simulink model "afe_abc_inv_pmsm"  (R2024b)
settings: Solver=ode1be  StartTime=0.0  StopTime=simlength  FixedStep=tc  MaxStep=tc
undefined symbols (not defined in the file): Adrso, Amplitude_U, Amplitude_V, Amplitude_W, Aresd, b, Bresd, Cresd, Crso, CTRPIFF_CLIP_RELEASE, dead_time_AFE, dead_time_INV, deepNEGeta, deepNEGxi, deepPOSxi, emf_fb_p, emf_fb_p_ccaller_1, emf_fb_p_ccaller_2, emf_p, emf_p_ccaller_1, emf_p_ccaller_2, end_time_LVRT, fPWM_AFE, fPWM_INV, g0_161Hz, g0_500Hz, g1_161Hz, g1_500Hz, i_grid_neg_eta_lim, i_grid_neg_eta_red_lim, i_grid_neg_xi_lim, i_grid_neg_xi_red_lim, i_grid_pos_eta_lim, i_grid_pos_eta_red_lim, ibez, id_lim, ieta_neg_ref_lim, ieta_pos_ref_lim, Igrid_phase_normalization_factor, iq_lim, ixi_pos_ref_lim, Jm, k_frt_ref, kg, ki_afe, ki_i, ki_rc_neg_grid, ki_rc_pos_grid, ki_vs, ki_w, kp_afe, kp_i, kp_rc_neg_grid, kp_rc_pos_grid, kp_vs, kp_w, kw, l1, l2, Ld_norm ... (+45)
libraries: fl_lib x115, nesl_utility x75, cstblocks x14, simulink x13, single_phase_transformer_lib x3, threephase_inductor_lib x2, flexshaft_lib x1, pmsm_uvw_with_harmonics_lib x1
(part 4 of 10)

== system afe_abc_inv_pmsm/afe_abc_inv_psm_mod1/inverter_control/torque_reference ==
  rotor speed : Inport
  1-D Lookup Table : Lookup_n-D  NumberOfTableDimensions=1  BreakpointsForDimension1=rpm_base  Table=torque_base  InternalRulePriority=Speed  RndMeth=Simplest
  Gain : Gain  Gain=-1
  Gain1 : Gain  Gain=1/tau_bez
  Gain2 : Gain  Gain=rpm_bez
  Saturation : Saturate  UpperLimit=0  LowerLimit=-inf
  Transfer Fcn : TransferFcn  Denominator=[1E-4 1]
  torque_ref : Outport
  wires:
  Transfer Fcn/1 -> Gain2/1
  rotor speed/1 -> Transfer Fcn/1
  Gain/1 -> Saturation/1
  Saturation/1 -> torque_ref/1
  Gain1/1 -> Gain/1
  1-D Lookup Table/1 -> Gain1/1
  Gain2/1 -> 1-D Lookup Table/1

== system afe_abc_inv_pmsm/grid/grid_emulator/3ph_Dyg ==
  Electrical Reference1 : fl_lib/Electrical/Electrical Elements/Electrical Reference
  ph1 : single_phase_transformer_lib/single phase transformer  Lm=Lmu2_trafo H  n1=50*sqrt(3)  n2=50  Rd1=0 Ohm  Rd2=Rd2_trafo Ohm  Ld1=0 H  Ld2=Ld2_trafo H  Rfe=Rm2_trafo Ohm  phi_specify=off  phi_priority=None  phi=0 V*s  phi_nominal_specify=off  phi_nominal_unit=V*s  phi_nominal_value=1  i1_specify=off  i1_priority=None  i1=0 A  i1_nominal_specify=off  i1_nominal_unit=A  i1_nominal_value=1  i2_specify=off  i2_priority=None  i2=0 A  i2_nominal_specify=off  i2_nominal_unit=A  i2_nominal_value=1  ife_specify=off  ife_priority=None  ife=0 A  ife_nominal_specify=off  ife_nominal_unit=A  ife_nominal_value=1  u1_specify=off  u1_priority=None  u1=0 V  u1_nominal_specify=off  u1_nominal_unit=V  u1_nominal_value=1  u2_specify=off  u2_priority=None  u2=0 V  u2_nominal_specify=off  u2_nominal_unit=V  u2_nominal_value=1
      settings: InternalSimscapePortConfiguration="{\"Bottom\":[],\"Left\":[{\"id\":\"u1_p\",\"label\":\"u1(+)\",\"type\":\"foundation.electrical.electrical\"},{\"id\":\"u1_n\",\"label\":\"u1(-)\",\"type\":\"foundation.electrical.electrical\"}],\"Right\":[{\"id\":\"u2_p\",\"label\":\"u2(+)\",\"type\":\"foundation.electrical.electrical\"},{\"id\":\"u2_n\",\"label\":\"u2(-)\",\"type\":\"foundation.electrical.electrical\"}],\"Top\":[]}"
  ph2 : single_phase_transformer_lib/single phase transformer  Lm=Lmu2_trafo H  n1=50*sqrt(3)  n2=50  Rd1=0 Ohm  Rd2=Rd2_trafo Ohm  Ld1=0 H  Ld2=Ld2_trafo H  Rfe=Rm2_trafo Ohm  phi_specify=off  phi_priority=None  phi=0 V*s  phi_nominal_specify=off  phi_nominal_unit=V*s  phi_nominal_value=1  i1_specify=off  i1_priority=None  i1=0 A  i1_nominal_specify=off  i1_nominal_unit=A  i1_nominal_value=1  i2_specify=off  i2_priority=None  i2=0 A  i2_nominal_specify=off  i2_nominal_unit=A  i2_nominal_value=1  ife_specify=off  ife_priority=None  ife=0 A  ife_nominal_specify=off  ife_nominal_unit=A  ife_nominal_value=1  u1_specify=off  u1_priority=None  u1=0 V  u1_nominal_specify=off  u1_nominal_unit=V  u1_nominal_value=1  u2_specify=off  u2_priority=None  u2=0 V  u2_nominal_specify=off  u2_nominal_unit=V  u2_nominal_value=1
      settings: InternalSimscapePortConfiguration="{\"Bottom\":[],\"Left\":[{\"id\":\"u1_p\",\"label\":\"u1(+)\",\"type\":\"foundation.electrical.electrical\"},{\"id\":\"u1_n\",\"label\":\"u1(-)\",\"type\":\"foundation.electrical.electrical\"}],\"Right\":[{\"id\":\"u2_p\",\"label\":\"u2(+)\",\"type\":\"foundation.electrical.electrical\"},{\"id\":\"u2_n\",\"label\":\"u2(-)\",\"type\":\"foundation.electrical.electrical\"}],\"Top\":[]}"
  ph3 : single_phase_transformer_lib/single phase transformer  Lm=Lmu2_trafo H  n1=50*sqrt(3)  n2=50  Rd1=0 Ohm  Rd2=Rd2_trafo Ohm  Ld1=0 H  Ld2=Ld2_trafo H  Rfe=Rm2_trafo Ohm  phi_specify=off  phi_priority=None  phi=0 V*s  phi_nominal_specify=off  phi_nominal_unit=V*s  phi_nominal_value=1  i1_specify=off  i1_priority=None  i1=0 A  i1_nominal_specify=off  i1_nominal_unit=A  i1_nominal_value=1  i2_specify=off  i2_priority=None  i2=0 A  i2_nominal_specify=off  i2_nominal_unit=A  i2_nominal_value=1  ife_specify=off  ife_priority=None  ife=0 A  ife_nominal_specify=off  ife_nominal_unit=A  ife_nominal_value=1  u1_specify=off  u1_priority=None  u1=0 V  u1_nominal_specify=off  u1_nominal_unit=V  u1_nominal_value=1  u2_specify=off  u2_priority=None  u2=0 V  u2_nominal_specify=off  u2_nominal_unit=V  u2_nominal_value=1
      settings: InternalSimscapePortConfiguration="{\"Bottom\":[],\"Left\":[{\"id\":\"u1_p\",\"label\":\"u1(+)\",\"type\":\"foundation.electrical.electrical\"},{\"id\":\"u1_n\",\"label\":\"u1(-)\",\"type\":\"foundation.electrical.electrical\"}],\"Right\":[{\"id\":\"u2_p\",\"label\":\"u2(+)\",\"type\":\"foundation.electrical.electrical\"},{\"id\":\"u2_n\",\"label\":\"u2(-)\",\"type\":\"foundation.electrical.electrical\"}],\"Top\":[]}"
  ua : PMIOPort  Side=Right
  ub : PMIOPort  Port=2  Side=Right
  uc : PMIOPort  Port=3  Side=Right
  Ua : PMIOPort  Port=4  Side=Left
  Ub : PMIOPort  Port=5  Side=Left
  Uc : PMIOPort  Port=6  Side=Left
  connections:
  Electrical Reference1/LConn1 -- ph3/RConn2 -- ph2/RConn2 -- ph1/RConn2
  ph3/RConn1 -- uc/RConn1
  ph1/LConn1 -- ph3/LConn2 -- Ua/RConn1
  ph1/RConn1 -- ua/RConn1
  ph2/RConn1 -- ub/RConn1
  ph1/LConn2 -- ph2/LConn1 -- Ub/RConn1
  Uc/RConn1 -- ph3/LConn1 -- ph2/LConn2

== system afe_abc_inv_pmsm/grid/grid_emulator/breaker ==
  PS Step : fl_lib/Physical Signals/Sources/PS Step  step_time=start_time_grid_switch_open s  initial_value=15  final_value=0
  switch_1 : Subsystem
      settings: PortSchema="{\"entries\":[{\"content\":{\"sides\":[{\"content\":{\"connectorIds\":[\"LConn1\"]},\"type\":\"ConnectorPlacement.EquallySpacedRectSide\",\"uuid\":\"9277da8d-d460-43e6-8478-dd662f15d226\"},{\"content\":{\"connectorIds\":[],\"side\":\"RIGHT\"},\"type\":\"ConnectorPlacement.EquallySpacedRectSide\",\"uuid\":\"a7ece396-f1d9-4f4f-a05b-db1fc65d6e1d\"},{\"content\":{\"connectorIds\":[\"LConn2\"],\"side\":\"TOP\"},\"type\":\"ConnectorPlacement.EquallySpacedRectSide\",\"uuid\":\"fdd70777-e9cf-4317-afb6-cae87f75d5b0\"},{\"content\":{\"connectorIds\":[\"RConn1\"],\"side\":\"BOTTOM\"},\"type\":\"ConnectorPlacement.EquallySpacedRectSide\",\"uuid\":\"2353ed68-b1a1-4775-9ca9-31e268d5443b\"}]},\"type\":\"ConnectorPlacement.EquallySpacedConnector\",\"uuid\":\"d5479f4c-4e65-4791-adcb-73df11f88590\"}],\"packageUris\":[\"http://schema.mathworks.com/mf0/Connector/R2020b\"],\"version\":\"1.0\"}"
  switch_2 : Subsystem
      settings: PortSchema="{\"entries\":[{\"content\":{\"sides\":[{\"content\":{\"connectorIds\":[\"LConn1\"]},\"type\":\"ConnectorPlacement.EquallySpacedRectSide\",\"uuid\":\"9277da8d-d460-43e6-8478-dd662f15d226\"},{\"content\":{\"connectorIds\":[],\"side\":\"RIGHT\"},\"type\":\"ConnectorPlacement.EquallySpacedRectSide\",\"uuid\":\"a7ece396-f1d9-4f4f-a05b-db1fc65d6e1d\"},{\"content\":{\"connectorIds\":[\"LConn2\"],\"side\":\"TOP\"},\"type\":\"ConnectorPlacement.EquallySpacedRectSide\",\"uuid\":\"fdd70777-e9cf-4317-afb6-cae87f75d5b0\"},{\"content\":{\"connectorIds\":[\"RConn1\"],\"side\":\"BOTTOM\"},\"type\":\"ConnectorPlacement.EquallySpacedRectSide\",\"uuid\":\"2353ed68-b1a1-4775-9ca9-31e268d5443b\"}]},\"type\":\"ConnectorPlacement.EquallySpacedConnector\",\"uuid\":\"d5479f4c-4e65-4791-adcb-73df11f88590\"}],\"packageUris\":[\"http://schema.mathworks.com/mf0/Connector/R2020b\"],\"version\":\"1.0\"}"
  switch_3 : Subsystem
      settings: PortSchema="{\"entries\":[{\"content\":{\"sides\":[{\"content\":{\"connectorIds\":[\"LConn1\"]},\"type\":\"ConnectorPlacement.EquallySpacedRectSide\",\"uuid\":\"9277da8d-d460-43e6-8478-dd662f15d226\"},{\"content\":{\"connectorIds\":[],\"side\":\"RIGHT\"},\"type\":\"ConnectorPlacement.EquallySpacedRectSide\",\"uuid\":\"a7ece396-f1d9-4f4f-a05b-db1fc65d6e1d\"},{\"content\":{\"connectorIds\":[\"LConn2\"],\"side\":\"TOP\"},\"type\":\"ConnectorPlacement.EquallySpacedRectSide\",\"uuid\":\"fdd70777-e9cf-4317-afb6-cae87f75d5b0\"},{\"content\":{\"connectorIds\":[\"RConn1\"],\"side\":\"BOTTOM\"},\"type\":\"ConnectorPlacement.EquallySpacedRectSide\",\"uuid\":\"2353ed68-b1a1-4775-9ca9-31e268d5443b\"}]},\"type\":\"ConnectorPlacement.EquallySpacedConnector\",\"uuid\":\"d5479f4c-4e65-4791-adcb-73df11f88590\"}],\"packageUris\":[\"http://schema.mathworks.com/mf0/Connector/R2020b\"],\"version\":\"1.0\"}"
  ua : PMIOPort  Side=Right
  Ua : PMIOPort  Port=2  Side=Left
  ub : PMIOPort  Port=3  Side=Right
  Ub : PMIOPort  Port=4  Side=Left
  uc : PMIOPort  Port=5  Side=Right
  Uc : PMIOPort  Port=6  Side=Left
  connections:
  Ub/RConn1 -- switch_2/LConn2
  Uc/RConn1 -- switch_3/LConn2
  Ua/RConn1 -- switch_1/LConn2
  PS Step/RConn1 -- switch_1/LConn1 -- switch_2/LConn1 -- switch_3/LConn1
  switch_1/RConn1 -- ua/RConn1
  ub/RConn1 -- switch_2/RConn1
  switch_3/RConn1 -- uc/RConn1

== system afe_abc_inv_pmsm/grid/grid_emulator/grid_emulator ==
  phase_gen : Subsystem
  voltage_reference : Subsystem
  voltage_source : Subsystem
  Vma : Outport
  Vmb : Outport  Port=2
  Vmc : Outport  Port=3
  wires:
  phase_gen/1(grid_emu_phase) -> voltage_reference/1(grid_emu_phase)  "grid_emu_phase"
  voltage_source/2(vn_xi) -> voltage_reference/3(Vxi_n)
  voltage_source/1(vp_xi) -> voltage_reference/2(Vxi_p)
  voltage_source/3(vn_eta) -> voltage_reference/4(Veta_n)
  voltage_reference/3(V3_ref) -> Vmc/1
  voltage_reference/1(V1_ref) -> Vma/1
  voltage_reference/2(V2_ref) -> Vmb/1

== system afe_abc_inv_pmsm/grid/grid_emulator/threephase_vi_measures ==
  Bus Creator : BusCreator  Inputs=6
  Current Sensor : fl_lib/Electrical/Electrical Sensors/Current Sensor
  Current Sensor1 : fl_lib/Electrical/Electrical Sensors/Current Sensor
  Current Sensor2 : fl_lib/Electrical/Electrical Sensors/Current Sensor
  Electrical Reference1 : fl_lib/Electrical/Electrical Elements/Electrical Reference
  Voltage Sensor : fl_lib/Electrical/Electrical Sensors/Voltage Sensor
  Voltage Sensor1 : fl_lib/Electrical/Electrical Sensors/Voltage Sensor
  Voltage Sensor2 : fl_lib/Electrical/Electrical Sensors/Voltage Sensor
  i : Selector  InputPortWidth=6  IndexOptions=Index vector (dialog)  Indices=[4 5 6]  OutputSizes=1
  i_line_abc/u_line_abc : Scope  NumInputPorts=2
  ia_grid : nesl_utility/PS-Simulink Converter  PhysicalDomain=network_engine_domain  SubClassName=ps_output  LeftPortType=input  RightPortType=output  PseudoPeriodic=off  Frequencies=[]  VectorFormat=1-D array  Unit=A  AffineConversion=off
  ib_grid : nesl_utility/PS-Simulink Converter  PhysicalDomain=network_engine_domain  SubClassName=ps_output  LeftPortType=input  RightPortType=output  PseudoPeriodic=off  Frequencies=[]  VectorFormat=1-D array  Unit=A  AffineConversion=off
  ic_grid : nesl_utility/PS-Simulink Converter  PhysicalDomain=network_engine_domain  SubClassName=ps_output  LeftPortType=input  RightPortType=output  PseudoPeriodic=off  Frequencies=[]  VectorFormat=1-D array  Unit=A  AffineConversion=off
  u : Selector  InputPortWidth=6  IndexOptions=Index vector (dialog)  Indices=[1 2 3]  OutputSizes=1
  ua_grid : nesl_utility/PS-Simulink Converter  PhysicalDomain=network_engine_domain  SubClassName=ps_output  LeftPortType=input  RightPortType=output  PseudoPeriodic=off  Frequencies=[]  VectorFormat=1-D array  Unit=V  AffineConversion=off
  ub_grid : nesl_utility/PS-Simulink Converter  PhysicalDomain=network_engine_domain  SubClassName=ps_output  LeftPortType=input  RightPortType=output  PseudoPeriodic=off  Frequencies=[]  VectorFormat=1-D array  Unit=V  AffineConversion=off
  uc_grid : nesl_utility/PS-Simulink Converter  PhysicalDomain=network_engine_domain  SubClassName=ps_output  LeftPortType=input  RightPortType=output  PseudoPeriodic=off  Frequencies=[]  VectorFormat=1-D array  Unit=V  AffineConversion=off
  Ua : PMIOPort  Side=Left
  ua : PMIOPort  Port=2  Side=Right
  Ub : PMIOPort  Port=3  Side=Left
  ub : PMIOPort  Port=4  Side=Right
  Uc : PMIOPort  Port=5  Side=Left
  uc : PMIOPort  Port=6  Side=Right
  wires:
  Bus Creator/1 -> i/1, u/1  "vi_data"
  ib_grid/1 -> Bus Creator/5  "ib"
  ia_grid/1 -> Bus Creator/4  "ia"
  ic_grid/1 -> Bus Creator/6  "ic"
  ua_grid/1 -> Bus Creator/1  "ua"
  ub_grid/1 -> Bus Creator/2  "ub"
  uc_grid/1 -> Bus Creator/3  "uc"
  i/1 -> i_line_abc/u_line_abc/1
  u/1 -> i_line_abc/u_line_abc/2
  connections:
  Current Sensor1/LConn1 -- Ub/RConn1 -- Voltage Sensor1/LConn1
  Electrical Reference1/LConn1 -- Voltage Sensor/RConn2 -- Voltage Sensor2/RConn2 -- Voltage Sensor1/RConn2
  Voltage Sensor/RConn1 -- ua_grid/LConn1
  Current Sensor/RConn2 -- ua/RConn1
  Voltage Sensor1/RConn1 -- ub_grid/LConn1
  Voltage Sensor2/LConn1 -- Current Sensor2/LConn1 -- Uc/RConn1
  Current Sensor/LConn1 -- Ua/RConn1 -- Voltage Sensor/LConn1
  Current Sensor1/RConn2 -- ub/RConn1
  Voltage Sensor2/RConn1 -- uc_grid/LConn1
  ib_grid/LConn1 -- Current Sensor1/RConn1
  ia_grid/LConn1 -- Current Sensor/RConn1
  ic_grid/LConn1 -- Current Sensor2/RConn1
  Current Sensor2/RConn2 -- uc/RConn1

== system afe_abc_inv_pmsm/grid/instantaneus_power/abc2alphabeta ==
  a : Inport
  b : Inport  Port=2
  c : Inport  Port=3
  abc2alphabeta : Subsystem
  vline_alpha : Outport  VectorParamsAs1DForOutWhenUnconnected=off
  vline_beta : Outport  Port=2  VectorParamsAs1DForOutWhenUnconnected=off
  wires:
  a/1 -> abc2alphabeta/1(a)
  b/1 -> abc2alphabeta/2(b)
  c/1 -> abc2alphabeta/3(c)
  abc2alphabeta/2("beta ") -> vline_beta/1
  abc2alphabeta/1("alpha ") -> vline_alpha/1

== system afe_abc_inv_pmsm/grid/instantaneus_power/abc2alphabeta  ==
  a : Inport
  b : Inport  Port=2
  c : Inport  Port=3
  abc->alphabeta : Subsystem
  i_line_alpha : Outport  VectorParamsAs1DForOutWhenUnconnected=off
  i_line_beta : Outport  Port=2  VectorParamsAs1DForOutWhenUnconnected=off
  wires:
  abc->alphabeta/1("alpha ") -> i_line_alpha/1
  abc->alphabeta/2("beta ") -> i_line_beta/1
  c/1 -> abc->alphabeta/3(c)
  b/1 -> abc->alphabeta/2(b)
  a/1 -> abc->alphabeta/1(a)

== system afe_abc_inv_pmsm/grid/instantaneus_power/moving_avarage ==
  In : Inport
  Gain1 : Gain  Gain=omega_grid_emulator_nom/2/pi  SaturateOnIntegerOverflow=on  OutDataTypeStr=Inherit: Same as input  ParamDataTypeStr=Inherit: Same as input
  Sum4 : Sum  SaturateOnIntegerOverflow=on
  Sum8 : Sum  Inputs=+-  InputSameDT=on  SaturateOnIntegerOverflow=on  OutDataTypeStr=Inherit: Same as first input
  Transport Delay : TransportDelay  DelayTime=2*pi/omega_grid_emulator_nom  BufferSize=2048*4  PadeOrder=2
  Unit Delay2 : UnitDelay  SampleTime=ts_afe  HasFrameUpgradeWarning=on
  kp2 : Gain  Gain=ts_afe  SaturateOnIntegerOverflow=on  OutDataTypeStr=Inherit: Same as input  ParamDataTypeStr=Inherit: Same as input
  Mean : Outport  VectorParamsAs1DForOutWhenUnconnected=off
  wires:
  Transport Delay/1 -> Sum8/2
  Sum4/1 -> Sum8/1, Transport Delay/1, Unit Delay2/1
  Sum8/1 -> Gain1/1
  In/1 -> kp2/1
  Unit Delay2/1 -> Sum4/2
  kp2/1 -> Sum4/1
  Gain1/1 -> Mean/1

== system afe_abc_inv_pmsm/grid/instantaneus_power/moving_avarage1 ==
  In : Inport
  Gain1 : Gain  Gain=omega_grid_emulator_nom/2/pi  SaturateOnIntegerOverflow=on  OutDataTypeStr=Inherit: Same as input  ParamDataTypeStr=Inherit: Same as input
  Sum4 : Sum  SaturateOnIntegerOverflow=on
  Sum8 : Sum  Inputs=+-  InputSameDT=on  SaturateOnIntegerOverflow=on  OutDataTypeStr=Inherit: Same as first input
  Transport Delay : TransportDelay  DelayTime=2*pi/omega_grid_emulator_nom  BufferSize=2048*4  PadeOrder=2
  Unit Delay2 : UnitDelay  SampleTime=ts_afe  HasFrameUpgradeWarning=on
  kp2 : Gain  Gain=ts_afe  SaturateOnIntegerOverflow=on  OutDataTypeStr=Inherit: Same as input  ParamDataTypeStr=Inherit: Same as input
  Mean : Outport  VectorParamsAs1DForOutWhenUnconnected=off
  wires:
  Gain1/1 -> Mean/1
  kp2/1 -> Sum4/1
  Unit Delay2/1 -> Sum4/2
  In/1 -> kp2/1
  Sum8/1 -> Gain1/1
  Sum4/1 -> Unit Delay2/1, Transport Delay/1, Sum8/1
  Transport Delay/1 -> Sum8/2

== system afe_abc_inv_pmsm/grid/instantaneus_power/rms ==
  In1 : Inport
  Gain : Gain  Gain=n10-1
  Gain1 : Gain  Gain=1/n10
  Math Function : Math  Operator=magnitude^2  SignedPower=on
  Sqrt : Sqrt
  Sum : Sum  Inputs=|++
  Unit Delay : UnitDelay  SampleTime=ts_afe  HasFrameUpgradeWarning=on
  Out1 : Outport  VectorParamsAs1DForOutWhenUnconnected=off
  wires:
  In1/1 -> Math Function/1
  Sum/1 -> Gain1/1
  Gain1/1 -> Sqrt/1, Unit Delay/1
  Unit Delay/1 -> Gain/1
  Math Function/1 -> Sum/1
  Sqrt/1 -> Out1/1
  Gain/1 -> Sum/2

== system afe_abc_inv_pmsm/grid/instantaneus_power/rms1 ==
  In1 : Inport
  Gain : Gain  Gain=n10-1
  Gain1 : Gain  Gain=1/n10
  Math Function : Math  Operator=magnitude^2  SignedPower=on
  Sqrt : Sqrt
  Sum : Sum  Inputs=|++
  Unit Delay : UnitDelay  SampleTime=ts_afe  HasFrameUpgradeWarning=on
  Out1 : Outport  VectorParamsAs1DForOutWhenUnconnected=off
  wires:
  Gain/1 -> Sum/2
  Sqrt/1 -> Out1/1
  Math Function/1 -> Sum/1
  Unit Delay/1 -> Gain/1
  Gain1/1 -> Unit Delay/1, Sqrt/1
  Sum/1 -> Gain1/1
  In1/1 -> Math Function/1

== system afe_abc_inv_pmsm/grid/instantaneus_power/rms2 ==
  In1 : Inport
  Gain : Gain  Gain=n10-1
  Gain1 : Gain  Gain=1/n10
  Math Function : Math  Operator=magnitude^2  SignedPower=on
  Sqrt : Sqrt
  Sum : Sum  Inputs=|++
  Unit Delay : UnitDelay  SampleTime=ts_afe  HasFrameUpgradeWarning=on
  Out1 : Outport  VectorParamsAs1DForOutWhenUnconnected=off
  wires:
  In1/1 -> Math Function/1
  Sum/1 -> Gain1/1
  Gain1/1 -> Sqrt/1, Unit Delay/1
  Unit Delay/1 -> Gain/1
  Math Function/1 -> Sum/1
  Sqrt/1 -> Out1/1
  Gain/1 -> Sum/2

== system afe_abc_inv_pmsm/grid/instantaneus_power/rms3 ==
  In1 : Inport
  Gain : Gain  Gain=n10-1
  Gain1 : Gain  Gain=1/n10
  Math Function : Math  Operator=magnitude^2  SignedPower=on
  Sqrt : Sqrt
  Sum : Sum  Inputs=|++
  Unit Delay : UnitDelay  SampleTime=ts_afe  HasFrameUpgradeWarning=on
  Out1 : Outport  VectorParamsAs1DForOutWhenUnconnected=off
  wires:
  Gain/1 -> Sum/2
  Sqrt/1 -> Out1/1
  Math Function/1 -> Sum/1
  Unit Delay/1 -> Gain/1
  Gain1/1 -> Unit Delay/1, Sqrt/1
  Sum/1 -> Gain1/1
  In1/1 -> Math Function/1

== system afe_abc_inv_pmsm/grid/instantaneus_power/rms4 ==
  In1 : Inport
  Gain : Gain  Gain=n10-1
  Gain1 : Gain  Gain=1/n10
  Math Function : Math  Operator=magnitude^2  SignedPower=on
  Sqrt : Sqrt
  Sum : Sum  Inputs=|++
  Unit Delay : UnitDelay  SampleTime=ts_afe  HasFrameUpgradeWarning=on
  Out1 : Outport  VectorParamsAs1DForOutWhenUnconnected=off
  wires:
  In1/1 -> Math Function/1
  Sum/1 -> Gain1/1
  Gain1/1 -> Sqrt/1, Unit Delay/1
  Unit Delay/1 -> Gain/1
  Math Function/1 -> Sum/1
  Sqrt/1 -> Out1/1
  Gain/1 -> Sum/2

== system afe_abc_inv_pmsm/grid/instantaneus_power/rms5 ==
  In1 : Inport
  Gain : Gain  Gain=n10-1
  Gain1 : Gain  Gain=1/n10
  Math Function : Math  Operator=magnitude^2  SignedPower=on
  Sqrt : Sqrt
  Sum : Sum  Inputs=|++
  Unit Delay : UnitDelay  SampleTime=ts_afe  HasFrameUpgradeWarning=on
  Out1 : Outport  VectorParamsAs1DForOutWhenUnconnected=off
  wires:
  Gain/1 -> Sum/2
  Sqrt/1 -> Out1/1
  Math Function/1 -> Sum/1
  Unit Delay/1 -> Gain/1
  Gain1/1 -> Unit Delay/1, Sqrt/1
  Sum/1 -> Gain1/1
  In1/1 -> Math Function/1

== system afe_abc_inv_pmsm/grid/sequences/moving_avarage ==
  In : Inport
  Gain1 : Gain  Gain=omega_grid_emulator_nom/2/pi  SaturateOnIntegerOverflow=on  OutDataTypeStr=Inherit: Same as input  ParamDataTypeStr=Inherit: Same as input
  Sum4 : Sum  SaturateOnIntegerOverflow=on
  Sum8 : Sum  Inputs=+-  InputSameDT=on  SaturateOnIntegerOverflow=on  OutDataTypeStr=Inherit: Same as first input
  Transport Delay : TransportDelay  DelayTime=2*pi/omega_grid_emulator_nom  BufferSize=2048*4  PadeOrder=2
  Unit Delay2 : UnitDelay  SampleTime=ts_afe  HasFrameUpgradeWarning=on
  kp2 : Gain  Gain=ts_afe  SaturateOnIntegerOverflow=on  OutDataTypeStr=Inherit: Same as input  ParamDataTypeStr=Inherit: Same as input
  Mean : Outport  VectorParamsAs1DForOutWhenUnconnected=off
  wires:
  Transport Delay/1 -> Sum8/2
  Sum4/1 -> Sum8/1, Transport Delay/1, Unit Delay2/1
  Sum8/1 -> Gain1/1
  In/1 -> kp2/1
  Unit Delay2/1 -> Sum4/2
  kp2/1 -> Sum4/1
  Gain1/1 -> Mean/1

== system afe_abc_inv_pmsm/grid/sequences/moving_avarage1 ==
  In : Inport
  Gain1 : Gain  Gain=omega_grid_emulator_nom/2/pi  SaturateOnIntegerOverflow=on  OutDataTypeStr=Inherit: Same as input  ParamDataTypeStr=Inherit: Same as input
  Sum4 : Sum  SaturateOnIntegerOverflow=on
  Sum8 : Sum  Inputs=+-  InputSameDT=on  SaturateOnIntegerOverflow=on  OutDataTypeStr=Inherit: Same as first input
  Transport Delay : TransportDelay  DelayTime=2*pi/omega_grid_emulator_nom  BufferSize=2048*4  PadeOrder=2
  Unit Delay2 : UnitDelay  SampleTime=ts_afe  HasFrameUpgradeWarning=on
  kp2 : Gain  Gain=ts_afe  SaturateOnIntegerOverflow=on  OutDataTypeStr=Inherit: Same as input  ParamDataTypeStr=Inherit: Same as input
  Mean : Outport  VectorParamsAs1DForOutWhenUnconnected=off
  wires:
  Gain1/1 -> Mean/1
  kp2/1 -> Sum4/1
  Unit Delay2/1 -> Sum4/2
  In/1 -> kp2/1
  Sum8/1 -> Gain1/1
  Sum4/1 -> Unit Delay2/1, Transport Delay/1, Sum8/1
  Transport Delay/1 -> Sum8/2

== system afe_abc_inv_pmsm/grid/sequences/moving_avarage10 ==
  In : Inport
  Gain1 : Gain  Gain=omega_grid_emulator_nom/2/pi  SaturateOnIntegerOverflow=on  OutDataTypeStr=Inherit: Same as input  ParamDataTypeStr=Inherit: Same as input
  Sum4 : Sum  SaturateOnIntegerOverflow=on
  Sum8 : Sum  Inputs=+-  InputSameDT=on  SaturateOnIntegerOverflow=on  OutDataTypeStr=Inherit: Same as first input
  Transport Delay : TransportDelay  DelayTime=2*pi/omega_grid_emulator_nom  BufferSize=2048*4  PadeOrder=2
  Unit Delay2 : UnitDelay  SampleTime=ts_afe  HasFrameUpgradeWarning=on
  kp2 : Gain  Gain=ts_afe  SaturateOnIntegerOverflow=on  OutDataTypeStr=Inherit: Same as input  ParamDataTypeStr=Inherit: Same as input
  Mean : Outport  VectorParamsAs1DForOutWhenUnconnected=off
  wires:
  Transport Delay/1 -> Sum8/2
  Sum4/1 -> Sum8/1, Transport Delay/1, Unit Delay2/1
  Sum8/1 -> Gain1/1
  In/1 -> kp2/1
  Unit Delay2/1 -> Sum4/2
  kp2/1 -> Sum4/1
  Gain1/1 -> Mean/1

== system afe_abc_inv_pmsm/grid/sequences/moving_avarage11 ==
  In : Inport
  Gain1 : Gain  Gain=omega_grid_emulator_nom/2/pi  SaturateOnIntegerOverflow=on  OutDataTypeStr=Inherit: Same as input  ParamDataTypeStr=Inherit: Same as input
  Sum4 : Sum  SaturateOnIntegerOverflow=on
  Sum8 : Sum  Inputs=+-  InputSameDT=on  SaturateOnIntegerOverflow=on  OutDataTypeStr=Inherit: Same as first input
  Transport Delay : TransportDelay  DelayTime=2*pi/omega_grid_emulator_nom  BufferSize=2048*4  PadeOrder=2
  Unit Delay2 : UnitDelay  SampleTime=ts_afe  HasFrameUpgradeWarning=on
  kp2 : Gain  Gain=ts_afe  SaturateOnIntegerOverflow=on  OutDataTypeStr=Inherit: Same as input  ParamDataTypeStr=Inherit: Same as input
  Mean : Outport  VectorParamsAs1DForOutWhenUnconnected=off
  wires:
  Gain1/1 -> Mean/1
  kp2/1 -> Sum4/1
  Unit Delay2/1 -> Sum4/2
  In/1 -> kp2/1
  Sum8/1 -> Gain1/1
  Sum4/1 -> Unit Delay2/1, Transport Delay/1, Sum8/1
  Transport Delay/1 -> Sum8/2

== system afe_abc_inv_pmsm/grid/sequences/moving_avarage2 ==
  In : Inport
  Gain1 : Gain  Gain=omega_grid_emulator_nom/2/pi  SaturateOnIntegerOverflow=on  OutDataTypeStr=Inherit: Same as input  ParamDataTypeStr=Inherit: Same as input
  Sum4 : Sum  SaturateOnIntegerOverflow=on
  Sum8 : Sum  Inputs=+-  InputSameDT=on  SaturateOnIntegerOverflow=on  OutDataTypeStr=Inherit: Same as first input
  Transport Delay : TransportDelay  DelayTime=2*pi/omega_grid_emulator_nom  BufferSize=2048*4  PadeOrder=2
  Unit Delay2 : UnitDelay  SampleTime=ts_afe  HasFrameUpgradeWarning=on
  kp2 : Gain  Gain=ts_afe  SaturateOnIntegerOverflow=on  OutDataTypeStr=Inherit: Same as input  ParamDataTypeStr=Inherit: Same as input
  Mean : Outport  VectorParamsAs1DForOutWhenUnconnected=off
  wires:
  Transport Delay/1 -> Sum8/2
  Sum4/1 -> Sum8/1, Transport Delay/1, Unit Delay2/1
  Sum8/1 -> Gain1/1
  In/1 -> kp2/1
  Unit Delay2/1 -> Sum4/2
  kp2/1 -> Sum4/1
  Gain1/1 -> Mean/1

== system afe_abc_inv_pmsm/grid/sequences/moving_avarage3 ==
  In : Inport
  Gain1 : Gain  Gain=omega_grid_emulator_nom/2/pi  SaturateOnIntegerOverflow=on  OutDataTypeStr=Inherit: Same as input  ParamDataTypeStr=Inherit: Same as input
  Sum4 : Sum  SaturateOnIntegerOverflow=on
  Sum8 : Sum  Inputs=+-  InputSameDT=on  SaturateOnIntegerOverflow=on  OutDataTypeStr=Inherit: Same as first input
  Transport Delay : TransportDelay  DelayTime=2*pi/omega_grid_emulator_nom  BufferSize=2048*4  PadeOrder=2
  Unit Delay2 : UnitDelay  SampleTime=ts_afe  HasFrameUpgradeWarning=on
  kp2 : Gain  Gain=ts_afe  SaturateOnIntegerOverflow=on  OutDataTypeStr=Inherit: Same as input  ParamDataTypeStr=Inherit: Same as input
  Mean : Outport  VectorParamsAs1DForOutWhenUnconnected=off
  wires:
  Gain1/1 -> Mean/1
  kp2/1 -> Sum4/1
  Unit Delay2/1 -> Sum4/2
  In/1 -> kp2/1
  Sum8/1 -> Gain1/1
  Sum4/1 -> Unit Delay2/1, Transport Delay/1, Sum8/1
  Transport Delay/1 -> Sum8/2

== system afe_abc_inv_pmsm/grid/sequences/moving_avarage4 ==
  In : Inport
  Gain1 : Gain  Gain=omega_grid_emulator_nom/2/pi  SaturateOnIntegerOverflow=on  OutDataTypeStr=Inherit: Same as input  ParamDataTypeStr=Inherit: Same as input
  Sum4 : Sum  SaturateOnIntegerOverflow=on
  Sum8 : Sum  Inputs=+-  InputSameDT=on  SaturateOnIntegerOverflow=on  OutDataTypeStr=Inherit: Same as first input
  Transport Delay : TransportDelay  DelayTime=2*pi/omega_grid_emulator_nom  BufferSize=2048*4  PadeOrder=2
  Unit Delay2 : UnitDelay  SampleTime=ts_afe  HasFrameUpgradeWarning=on
  kp2 : Gain  Gain=ts_afe  SaturateOnIntegerOverflow=on  OutDataTypeStr=Inherit: Same as input  ParamDataTypeStr=Inherit: Same as input
  Mean : Outport  VectorParamsAs1DForOutWhenUnconnected=off
  wires:
  Transport Delay/1 -> Sum8/2
  Sum4/1 -> Sum8/1, Transport Delay/1, Unit Delay2/1
  Sum8/1 -> Gain1/1
  In/1 -> kp2/1
  Unit Delay2/1 -> Sum4/2
  kp2/1 -> Sum4/1
  Gain1/1 -> Mean/1

== system afe_abc_inv_pmsm/grid/sequences/moving_avarage5 ==
  In : Inport
  Gain1 : Gain  Gain=omega_grid_emulator_nom/2/pi  SaturateOnIntegerOverflow=on  OutDataTypeStr=Inherit: Same as input  ParamDataTypeStr=Inherit: Same as input
  Sum4 : Sum  SaturateOnIntegerOverflow=on
  Sum8 : Sum  Inputs=+-  InputSameDT=on  SaturateOnIntegerOverflow=on  OutDataTypeStr=Inherit: Same as first input
  Transport Delay : TransportDelay  DelayTime=2*pi/omega_grid_emulator_nom  BufferSize=2048*4  PadeOrder=2
  Unit Delay2 : UnitDelay  SampleTime=ts_afe  HasFrameUpgradeWarning=on
  kp2 : Gain  Gain=ts_afe  SaturateOnIntegerOverflow=on  OutDataTypeStr=Inherit: Same as input  ParamDataTypeStr=Inherit: Same as input
  Mean : Outport  VectorParamsAs1DForOutWhenUnconnected=off
  wires:
  Gain1/1 -> Mean/1
  kp2/1 -> Sum4/1
  Unit Delay2/1 -> Sum4/2
  In/1 -> kp2/1
  Sum8/1 -> Gain1/1
  Sum4/1 -> Unit Delay2/1, Transport Delay/1, Sum8/1
  Transport Delay/1 -> Sum8/2

== system afe_abc_inv_pmsm/grid/sequences/moving_avarage6 ==
  In : Inport
  Gain1 : Gain  Gain=omega_grid_emulator_nom/2/pi  SaturateOnIntegerOverflow=on  OutDataTypeStr=Inherit: Same as input  ParamDataTypeStr=Inherit: Same as input
  Sum4 : Sum  SaturateOnIntegerOverflow=on
  Sum8 : Sum  Inputs=+-  InputSameDT=on  SaturateOnIntegerOverflow=on  OutDataTypeStr=Inherit: Same as first input
  Transport Delay : TransportDelay  DelayTime=2*pi/omega_grid_emulator_nom  BufferSize=2048*4  PadeOrder=2
  Unit Delay2 : UnitDelay  SampleTime=ts_afe  HasFrameUpgradeWarning=on
  kp2 : Gain  Gain=ts_afe  SaturateOnIntegerOverflow=on  OutDataTypeStr=Inherit: Same as input  ParamDataTypeStr=Inherit: Same as input
  Mean : Outport  VectorParamsAs1DForOutWhenUnconnected=off
  wires:
  Transport Delay/1 -> Sum8/2
  Sum4/1 -> Sum8/1, Transport Delay/1, Unit Delay2/1
  Sum8/1 -> Gain1/1
  In/1 -> kp2/1
  Unit Delay2/1 -> Sum4/2
  kp2/1 -> Sum4/1
  Gain1/1 -> Mean/1

== system afe_abc_inv_pmsm/grid/sequences/moving_avarage7 ==
  In : Inport
  Gain1 : Gain  Gain=omega_grid_emulator_nom/2/pi  SaturateOnIntegerOverflow=on  OutDataTypeStr=Inherit: Same as input  ParamDataTypeStr=Inherit: Same as input
  Sum4 : Sum  SaturateOnIntegerOverflow=on
  Sum8 : Sum  Inputs=+-  InputSameDT=on  SaturateOnIntegerOverflow=on  OutDataTypeStr=Inherit: Same as first input
  Transport Delay : TransportDelay  DelayTime=2*pi/omega_grid_emulator_nom  BufferSize=2048*4  PadeOrder=2
  Unit Delay2 : UnitDelay  SampleTime=ts_afe  HasFrameUpgradeWarning=on
  kp2 : Gain  Gain=ts_afe  SaturateOnIntegerOverflow=on  OutDataTypeStr=Inherit: Same as input  ParamDataTypeStr=Inherit: Same as input
  Mean : Outport  VectorParamsAs1DForOutWhenUnconnected=off
  wires:
  Gain1/1 -> Mean/1
  kp2/1 -> Sum4/1
  Unit Delay2/1 -> Sum4/2
  In/1 -> kp2/1
  Sum8/1 -> Gain1/1
  Sum4/1 -> Unit Delay2/1, Transport Delay/1, Sum8/1
  Transport Delay/1 -> Sum8/2

== system afe_abc_inv_pmsm/grid/sequences/moving_avarage8 ==
  In : Inport
  Gain1 : Gain  Gain=omega_grid_emulator_nom/2/pi  SaturateOnIntegerOverflow=on  OutDataTypeStr=Inherit: Same as input  ParamDataTypeStr=Inherit: Same as input
  Sum4 : Sum  SaturateOnIntegerOverflow=on
  Sum8 : Sum  Inputs=+-  InputSameDT=on  SaturateOnIntegerOverflow=on  OutDataTypeStr=Inherit: Same as first input
  Transport Delay : TransportDelay  DelayTime=2*pi/omega_grid_emulator_nom  BufferSize=2048*4  PadeOrder=2
  Unit Delay2 : UnitDelay  SampleTime=ts_afe  HasFrameUpgradeWarning=on
  kp2 : Gain  Gain=ts_afe  SaturateOnIntegerOverflow=on  OutDataTypeStr=Inherit: Same as input  ParamDataTypeStr=Inherit: Same as input
  Mean : Outport  VectorParamsAs1DForOutWhenUnconnected=off
  wires:
  Transport Delay/1 -> Sum8/2
  Sum4/1 -> Sum8/1, Transport Delay/1, Unit Delay2/1
  Sum8/1 -> Gain1/1
  In/1 -> kp2/1
  Unit Delay2/1 -> Sum4/2
  kp2/1 -> Sum4/1
  Gain1/1 -> Mean/1

== system afe_abc_inv_pmsm/grid/sequences/moving_avarage9 ==
  In : Inport
  Gain1 : Gain  Gain=omega_grid_emulator_nom/2/pi  SaturateOnIntegerOverflow=on  OutDataTypeStr=Inherit: Same as input  ParamDataTypeStr=Inherit: Same as input
  Sum4 : Sum  SaturateOnIntegerOverflow=on
  Sum8 : Sum  Inputs=+-  InputSameDT=on  SaturateOnIntegerOverflow=on  OutDataTypeStr=Inherit: Same as first input
  Transport Delay : TransportDelay  DelayTime=2*pi/omega_grid_emulator_nom  BufferSize=2048*4  PadeOrder=2
  Unit Delay2 : UnitDelay  SampleTime=ts_afe  HasFrameUpgradeWarning=on
  kp2 : Gain  Gain=ts_afe  SaturateOnIntegerOverflow=on  OutDataTypeStr=Inherit: Same as input  ParamDataTypeStr=Inherit: Same as input
  Mean : Outport  VectorParamsAs1DForOutWhenUnconnected=off
  wires:
  Gain1/1 -> Mean/1
  kp2/1 -> Sum4/1
  Unit Delay2/1 -> Sum4/2
  In/1 -> kp2/1
  Sum8/1 -> Gain1/1
  Sum4/1 -> Unit Delay2/1, Transport Delay/1, Sum8/1
  Transport Delay/1 -> Sum8/2

== system afe_abc_inv_pmsm/afe_abc_inv_psm_mod1/afe/dclink_measure/R_derating ==
  Step : Step  After=107.4e3/2  SampleTime=0
  Step1 : Step  Time=1.1  After=-107.4e3/2  SampleTime=0
  Sum : Sum  Inputs=|++
  DR : Outport
  wires:
  Step1/1 -> Sum/2
  Step/1 -> Sum/1
  Sum/1 -> DR/1

== system afe_abc_inv_pmsm/afe_abc_inv_psm_mod1/afe/sv_pwm/modulator1 ==
  u : Inport
  v : Inport  Port=2
  w : Inport  Port=3
  phase : Inport  Port=4
  Bus Creator3 : BusCreator  Inputs=6
  PWM generator 1 : Subsystem  mask{f=fPWM_AFE, m_up=0.98, m_low=0.02, dead_time=dead_time_AFE, pos_cmd_gate=15, neg_cmd_gate=-10, polarity=1}
      mask prompts: f "Frequency (Hz)"; m_up "Max Input Modulation Value"; m_low "Min Input Modulation Value"; dead_time "Dead Time (s)"; pos_cmd_gate "Positive Gate Voltage (V)"; neg_cmd_gate "Negative Gate Voltage (V)"; polarity "Polarity (pu)"
  PWM generator 2 : Subsystem  mask{f=fPWM_AFE, m_up=0.98, m_low=0.02, dead_time=dead_time_AFE, pos_cmd_gate=15, neg_cmd_gate=-10, polarity=1}
      mask prompts: f "Frequency (Hz)"; m_up "Max Input Modulation Value"; m_low "Min Input Modulation Value"; dead_time "Dead Time (s)"; pos_cmd_gate "Positive Gate Voltage (V)"; neg_cmd_gate "Negative Gate Voltage (V)"; polarity "Polarity (pu)"
  PWM generator 3 : Subsystem  mask{f=fPWM_AFE, m_up=0.98, m_low=0.02, dead_time=dead_time_AFE, pos_cmd_gate=15, neg_cmd_gate=-10, polarity=1}
      mask prompts: f "Frequency (Hz)"; m_up "Max Input Modulation Value"; m_low "Min Input Modulation Value"; dead_time "Dead Time (s)"; pos_cmd_gate "Positive Gate Voltage (V)"; neg_cmd_gate "Negative Gate Voltage (V)"; polarity "Polarity (pu)"
  cmd_gates : Outport
  wires:
  u/1 -> PWM generator 1/1(m_index)
  w/1 -> PWM generator 3/1(m_index)
  v/1 -> PWM generator 2/1(m_index)
  phase/1 -> PWM generator 3/2(phase), PWM generator 2/2(phase), PWM generator 1/2(phase)
  PWM generator 1/2(m2) -> Bus Creator3/2  "pwm_afe_phase_u_bottom"
  PWM generator 3/1(m1) -> Bus Creator3/5  "pwm_afe_phase_w_top"
  PWM generator 2/1(m1) -> Bus Creator3/3  "pwm_afe_phase_v_top"
  PWM generator 2/2(m2) -> Bus Creator3/4  "pwm_afe_phase_v_bottom"
  PWM generator 3/2(m2) -> Bus Creator3/6  "pwm_afe_phase_w_bottom"
  PWM generator 1/1(m1) -> Bus Creator3/1  "pwm_afe_phase_u_top"
  Bus Creator3/1 -> cmd_gates/1

== system afe_abc_inv_pmsm/afe_abc_inv_psm_mod1/afe_control/current_ctrl/Inner Loop Current Control ==
  In1 : Inport
  is_abc : Inport  Port=2
  -1<x<1 : Saturate  UpperLimit=1  LowerLimit=-1
  Add : Sum
  Bus Creator1 : BusCreator  Inputs=2
  "Current-Control, Phase a" : Subsystem
  "Current-Control, Phase b" : Subsystem
  "Current-Control, Phase c" : Subsystem
  Demux1 : Demux  Outputs=3
  MATLAB Function : MATLAB Function  TreatAsAtomicUnit=on
  Mux : Mux  Inputs=3
  Selector : Selector  InputPortWidth=3  IndexOptions=Index vector (dialog)  Indices=[1]  OutputSizes=1
  Selector1 : Selector  InputPortWidth=3  IndexOptions=Index vector (dialog)  Indices=[1]  OutputSizes=1
  Selector2 : Selector  InputPortWidth=3  IndexOptions=Index vector (dialog)  Indices=[2]  OutputSizes=1
  Selector3 : Selector  InputPortWidth=3  IndexOptions=Index vector (dialog)  Indices=[2]  OutputSizes=1
  Selector4 : Selector  InputPortWidth=3  IndexOptions=Index vector (dialog)  Indices=[3]  OutputSizes=1
  Selector5 : Selector  InputPortWidth=3  IndexOptions=Index vector (dialog)  Indices=[3]  OutputSizes=1
  Unit Delay1 : UnitDelay  SampleTime=ts_afe  HasFrameUpgradeWarning=on
  Unit Delay2 : UnitDelay  SampleTime=ts_afe  HasFrameUpgradeWarning=on
  Unit Delay3 : UnitDelay  SampleTime=ts_afe  HasFrameUpgradeWarning=on
  isa_ref/isa : Scope  NumInputPorts=2
  isb_ref/isb : Scope  NumInputPorts=2
  isc_ref/isc : Scope  NumInputPorts=2
  uab : Outport  VectorParamsAs1DForOutWhenUnconnected=off
  wires:
  In1/1 -> Selector4/1, Selector2/1, Selector/1  "i_abc_ref"
  is_abc/1 -> Selector5/1, Selector3/1, Selector1/1  "i_abc"
  Add/1 -> -1<x<1/1  "v_abc"
  Selector/1 -> isa_ref/isa/1, "Current-Control, Phase a"/1(In1)  "isa_ref"
  Selector1/1 -> isa_ref/isa/2, "Current-Control, Phase a"/2(In2)  "isa"
  Selector2/1 -> isb_ref/isb/1, "Current-Control, Phase b"/1(In1)  "isb_ref"
  Selector3/1 -> isb_ref/isb/2, "Current-Control, Phase b"/2(In2)  "isb"
  Selector4/1 -> isc_ref/isc/1, "Current-Control, Phase c"/1(In1)  "isc_ref"
  Selector5/1 -> isc_ref/isc/2, "Current-Control, Phase c"/2(In2)  "isc"
  "Current-Control, Phase a"/1(Out1) -> Mux/1  "v_a"
  "Current-Control, Phase b"/1(Out1) -> Mux/2  "v_b"
  "Current-Control, Phase c"/1(Out1) -> Mux/3  "v_c"
  Mux/1 -> Add/1  "v_abc"
  [v_grid_ff_abc] -> Unit Delay1/1
  Demux1/3 -> MATLAB Function/3(c)  "v_c"
  MATLAB Function/1(alpha) -> Unit Delay2/1  "u_alpha"
  Unit Delay3/1 -> Bus Creator1/2  "ubeta_afe"
  Demux1/2 -> MATLAB Function/2(b)  "v_b"
  MATLAB Function/2(beta) -> Unit Delay3/1  "u_beta"
  Demux1/1 -> MATLAB Function/1(a)  "v_a"
  Unit Delay2/1 -> Bus Creator1/1  "ualpha_afe"
  Bus Creator1/1 -> uab/1
  -1<x<1/1 -> Demux1/1  "v_abc"
  Unit Delay1/1 -> Add/2

== system afe_abc_inv_pmsm/afe_abc_inv_psm_mod1/afe_control/current_ctrl/current_transformation ==
  is_a_pu : Inport
  is_b_pu : Inport  Port=2
  is_c_pu : Inport  Port=3
  Bus Creator : BusCreator  Inputs=3
  alphabeta2xieta : MATLAB Function  TreatAsAtomicUnit=on  SystemSampleTime=ts_afe
  uvw2alphabeta : MATLAB Function  TreatAsAtomicUnit=on  SystemSampleTime=ts_afe
  tag scope: i_eta_pu=global, i_xi_pu=global, is_abc_pu=global
  wires:
  is_c_pu/1 -> Bus Creator/3, uvw2alphabeta/3(w)
  alphabeta2xieta/2(eta) -> [i_eta_pu]  "ieta_pu"
  alphabeta2xieta/1(xi) -> [i_xi_pu]  "ixi_pu"
  is_b_pu/1 -> Bus Creator/2, uvw2alphabeta/2(v)
  uvw2alphabeta/2(beta) -> alphabeta2xieta/2(beta)  "ibeta_pu"
  uvw2alphabeta/1(alpha) -> alphabeta2xieta/1(alpha)  "ialpha_pu"
  [gamma_grid_pll] -> alphabeta2xieta/3(gamma)
  is_a_pu/1 -> Bus Creator/1, uvw2alphabeta/1(u)
  Bus Creator/1 -> [is_abc_pu]

== system afe_abc_inv_pmsm/afe_abc_inv_psm_mod1/afe_control/current_ctrl/sample_hold_normalization ==
  is_a : Inport
  is_b : Inport  Port=2
  is_c : Inport  Port=3
  Gain : Gain  Gain=1/Igrid_phase_normalization_factor
  Gain1 : Gain  Gain=1/Igrid_phase_normalization_factor
  Gain2 : Gain  Gain=1/Igrid_phase_normalization_factor
  Quantizer : Quantizer  QuantizationInterval=CurrentQuantization
  Quantizer1 : Quantizer  QuantizationInterval=CurrentQuantization
  Quantizer2 : Quantizer  QuantizationInterval=CurrentQuantization
  Unit Delay : UnitDelay  SampleTime=ts_afe  HasFrameUpgradeWarning=on
  Unit Delay1 : UnitDelay  SampleTime=ts_afe  HasFrameUpgradeWarning=on
  Unit Delay2 : UnitDelay  SampleTime=ts_afe  HasFrameUpgradeWarning=on
  Zero-Order Hold : ZeroOrderHold  SampleTime=ts_afe
  Zero-Order Hold1 : ZeroOrderHold  SampleTime=ts_afe
  Zero-Order Hold2 : ZeroOrderHold  SampleTime=ts_afe
  is_a_pu : Outport
  is_b_pu : Outport  Port=2
  is_c_pu : Outport  Port=3
  wires:
  is_a/1 -> Quantizer/1
  Unit Delay/1 -> Gain/1
  Zero-Order Hold/1 -> Unit Delay/1
  is_c/1 -> Quantizer2/1
  is_b/1 -> Quantizer1/1
  Gain/1 -> is_a_pu/1
  Gain1/1 -> is_b_pu/1
  Gain2/1 -> is_c_pu/1
  Unit Delay1/1 -> Gain1/1
  Unit Delay2/1 -> Gain2/1
  Zero-Order Hold1/1 -> Unit Delay1/1
  Zero-Order Hold2/1 -> Unit Delay2/1
  Quantizer/1 -> Zero-Order Hold/1
  Quantizer1/1 -> Zero-Order Hold1/1
  Quantizer2/1 -> Zero-Order Hold2/1

== system afe_abc_inv_pmsm/afe_abc_inv_psm_mod1/afe_control/current_ctrl/xieta2abc ==
  pos_xi : Inport
  pos_eta : Inport  Port=2
  neg_xi : Inport  Port=3
  neg_eta : Inport  Port=4
  gamma : Inport  Port=5
  MATLAB Function2 : MATLAB Function  TreatAsAtomicUnit=on
  Mux : Mux  Inputs=3
  Negative Sequence : MATLAB Function  TreatAsAtomicUnit=on
  Positive Sequence : MATLAB Function  TreatAsAtomicUnit=on
  Sum : Sum  Inputs=|++
  Sum1 : Sum  Inputs=|++
  i_abc : Outport
  wires:
  neg_eta/1 -> Negative Sequence/2(eta)
  MATLAB Function2/1(a) -> Mux/1  "i_a"
  Positive Sequence/2(beta) -> Sum1/1
  Sum/1 -> MATLAB Function2/1(alpha)
  gamma/1 -> Negative Sequence/3(gamma), Positive Sequence/3(gamma)
  MATLAB Function2/3(c) -> Mux/3  "i_c"
  Negative Sequence/1(alpha) -> Sum/2
  Positive Sequence/1(alpha) -> Sum/1
  Negative Sequence/2(beta) -> Sum1/2
  MATLAB Function2/2(b) -> Mux/2  "i_b"
  Sum1/1 -> MATLAB Function2/2(beta)
  neg_xi/1 -> Negative Sequence/1(xi)
  pos_xi/1 -> Positive Sequence/1(xi)
  pos_eta/1 -> Positive Sequence/2(eta)
  Mux/1 -> i_abc/1  "i_abc"

== system afe_abc_inv_pmsm/afe_abc_inv_psm_mod1/afe_control/current_sequence_avg/average_filter_ccaller ==
  i_grid_pos_xi : Inport
  i_grid_pos_eta : Inport  Port=2
  i_grid_neg_xi : Inport  Port=3
  i_grid_neg_eta : Inport  Port=4
  Moving Average Filter5 : Subsystem
  Moving Average Filter6 : Subsystem
  Moving Average Filter7 : Subsystem
  Moving Average Filter8 : Subsystem
  i_grid_pos_xi_avg : Outport
  i_grid_pos_eta_avg : Outport  Port=2
  i_grid_neg_xi_avg : Outport  Port=3
  i_grid_neg_eta_avg : Outport  Port=4
  wires:
  Moving Average Filter6/1(xi) -> i_grid_pos_eta_avg/1
  [omega_grid_pll] -> Moving Average Filter6/2(In3), Moving Average Filter8/2(In3), Moving Average Filter7/2(In3), Moving Average Filter5/2(In3)
  i_grid_pos_eta/1 -> Moving Average Filter6/1(In2)
  Moving Average Filter8/1(xi) -> i_grid_neg_eta_avg/1
  i_grid_neg_xi/1 -> Moving Average Filter7/1(In2)
  Moving Average Filter7/1(xi) -> i_grid_neg_xi_avg/1
  i_grid_pos_xi/1 -> Moving Average Filter5/1(In2)
  i_grid_neg_eta/1 -> Moving Average Filter8/1(In2)
  Moving Average Filter5/1(xi) -> i_grid_pos_xi_avg/1

== system afe_abc_inv_pmsm/afe_abc_inv_psm_mod1/afe_control/current_sequence_avg/average_filter_simulink ==
  i_grid_pos_xi : Inport
  i_grid_pos_eta : Inport  Port=2
  i_grid_neg_xi : Inport  Port=3
  i_grid_neg_eta : Inport  Port=4
  moving_avarage1 : Subsystem
  moving_avarage2 : Subsystem
  moving_avarage3 : Subsystem
  moving_avarage4 : Subsystem
  i_grid_pos_xi_avg : Outport
  i_grid_pos_eta_avg : Outport  Port=2
  i_grid_neg_xi_avg : Outport  Port=3
  i_grid_neg_eta_avg : Outport  Port=4
  wires:
  moving_avarage3/1(Mean) -> i_grid_neg_xi_avg/1
  moving_avarage1/1(Mean) -> i_grid_pos_xi_avg/1
  i_grid_pos_eta/1 -> moving_avarage2/1(In)
  i_grid_neg_eta/1 -> moving_avarage4/1(In)
  i_grid_pos_xi/1 -> moving_avarage1/1(In)
  moving_avarage4/1(Mean) -> i_grid_neg_eta_avg/1
  i_grid_neg_xi/1 -> moving_avarage3/1(In)
  moving_avarage2/1(Mean) -> i_grid_pos_eta_avg/1

== system afe_abc_inv_pmsm/afe_abc_inv_psm_mod1/afe_control/grid_current_sampling_and_alpha_beta_transformation/sample_hold_normalization ==
  ig_a : Inport
  ig_b : Inport  Port=2
  ig_c : Inport  Port=3
  Gain : Gain  Gain=1/Igrid_phase_normalization_factor
  Gain1 : Gain  Gain=1/Igrid_phase_normalization_factor
  Gain2 : Gain  Gain=1/Igrid_phase_normalization_factor
  Quantizer : Quantizer  QuantizationInterval=CurrentQuantization
  Quantizer1 : Quantizer  QuantizationInterval=CurrentQuantization
  Quantizer2 : Quantizer  QuantizationInterval=CurrentQuantization
  Unit Delay : UnitDelay  SampleTime=ts_afe  HasFrameUpgradeWarning=on
  Unit Delay1 : UnitDelay  SampleTime=ts_afe  HasFrameUpgradeWarning=on
  Unit Delay2 : UnitDelay  SampleTime=ts_afe  HasFrameUpgradeWarning=on
  Zero-Order Hold : ZeroOrderHold  SampleTime=ts_afe
  Zero-Order Hold1 : ZeroOrderHold  SampleTime=ts_afe
  Zero-Order Hold2 : ZeroOrderHold  SampleTime=ts_afe
  ig_a_pu : Outport
  ig_b_pu : Outport  Port=2
  ig_c_pu : Outport  Port=3
  wires:
  ig_a/1 -> Quantizer/1
  Unit Delay/1 -> Gain/1
  Zero-Order Hold/1 -> Unit Delay/1
  ig_c/1 -> Quantizer2/1
  ig_b/1 -> Quantizer1/1
  Gain/1 -> ig_a_pu/1
  Gain1/1 -> ig_b_pu/1
  Gain2/1 -> ig_c_pu/1
  Unit Delay1/1 -> Gain1/1
  Unit Delay2/1 -> Gain2/1
  Zero-Order Hold1/1 -> Unit Delay1/1
  Zero-Order Hold2/1 -> Unit Delay2/1
  Quantizer/1 -> Zero-Order Hold/1
  Quantizer1/1 -> Zero-Order Hold1/1
  Quantizer2/1 -> Zero-Order Hold2/1

== system afe_abc_inv_pmsm/afe_abc_inv_psm_mod1/afe_control/grid_voltage_phase_lock_loops/DDSRF-PLL ==
  pll_stageA : Subsystem
  pll_stageB : Subsystem
  grid_phase_out : Outport
  wires:
  pll_stageB/1(wt_grid) -> pll_stageA/1(gamma_grid), grid_phase_out/1
  pll_stageA/2(u_grid_pos_eta) -> pll_stageB/2(u_grid_pos_eta)  "u_grid_pos_eta"
  pll_stageA/1(u_grid_pos_xi) -> pll_stageB/1(u_grid_pos_xi)  "u_grid_pos_xi"

== system afe_abc_inv_pmsm/afe_abc_inv_psm_mod1/afe_control/grid_voltage_phase_lock_loops/DQ-PLL ==
  pll_stageA : Subsystem
  pll_stageB : Subsystem
  grid_phase_out : Outport
  wires:
  pll_stageA/2(u_grid_pos_eta) -> pll_stageB/2(u_grid_pos_eta)  "u_grid_pos_eta"
  pll_stageB/1(gamma_grid_pll) -> pll_stageA/1(gamma_grid), grid_phase_out/1
  pll_stageA/1(u_grid_pos_xi) -> pll_stageB/1(u_grid_pos_xi)  "u_grid_pos_xi"

== system afe_abc_inv_pmsm/afe_abc_inv_psm_mod1/afe_control/grid_voltage_sampling_and_alpha_beta_transformation/sample_hold_normalization ==
  vg_a : Inport
  vg_b : Inport  Port=2
  vg_c : Inport  Port=3
  Gain : Gain  Gain=1/Vgrid_phase_normalization_factor
  Gain1 : Gain  Gain=1/Vgrid_phase_normalization_factor
  Gain2 : Gain  Gain=1/Vgrid_phase_normalization_factor
  Quantizer1 : Quantizer  QuantizationInterval=VoltageQuantization
  Quantizer2 : Quantizer  QuantizationInterval=VoltageQuantization
  Quantizer3 : Quantizer  QuantizationInterval=VoltageQuantization
  Unit Delay : UnitDelay  SampleTime=ts_afe  HasFrameUpgradeWarning=on
  Unit Delay1 : UnitDelay  SampleTime=ts_afe  HasFrameUpgradeWarning=on
  Unit Delay2 : UnitDelay  SampleTime=ts_afe  HasFrameUpgradeWarning=on
  Zero-Order Hold : ZeroOrderHold  SampleTime=ts_afe
  Zero-Order Hold1 : ZeroOrderHold  SampleTime=ts_afe
  Zero-Order Hold2 : ZeroOrderHold  SampleTime=ts_afe
  vg_a_pu : Outport
  vg_b_pu : Outport  Port=2
  vg_c_pu : Outport  Port=3
  wires:
  vg_a/1 -> Quantizer1/1
  Unit Delay/1 -> Gain/1
  Zero-Order Hold/1 -> Unit Delay/1
  vg_c/1 -> Quantizer3/1
  vg_b/1 -> Quantizer2/1
  Gain/1 -> vg_a_pu/1
  Gain1/1 -> vg_b_pu/1
  Gain2/1 -> vg_c_pu/1
  Unit Delay1/1 -> Gain1/1
  Unit Delay2/1 -> Gain2/1
  Zero-Order Hold1/1 -> Unit Delay1/1
  Zero-Order Hold2/1 -> Unit Delay2/1
  Quantizer1/1 -> Zero-Order Hold/1
  Quantizer2/1 -> Zero-Order Hold1/1
  Quantizer3/1 -> Zero-Order Hold2/1
